simulink model "TestRtrIkslx"  (R2020a)
settings: Solver=VariableStepAuto  StartTime=0.0  StopTime=10.0  RelTol=1e-3
values from neighbouring files (symbols this model uses):
  l2 = 0.3    [TestingIkRTR.m]    (also in TestingScriptRTR.m)
  l3 = 0.2    [TestingIkRTR.m]    (also in TestingScriptRTR.m)
settings Model: Creator=ja  LastModifiedBy=ja

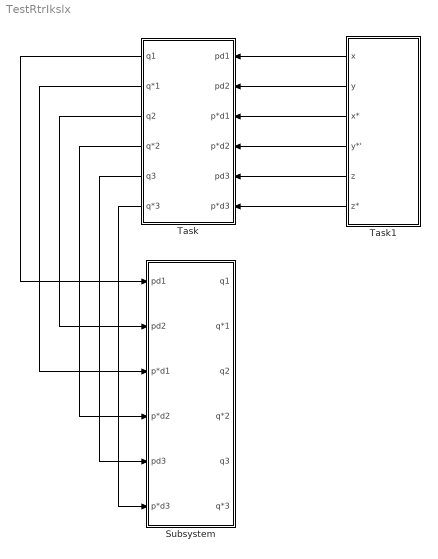
== system TestRtrIkslx ==
  Subsystem : Subsystem
  Task : Subsystem
  Task1 : Subsystem
  wires:
  Task1/5(z) -> Task/5(pd3)
  Task1/6(z*) -> Task/6(p*d3)
  Task1/1(x) -> Task/1(pd1)
  Task1/2(y) -> Task/2(pd2)
  Task1/3(x*) -> Task/3(p*d1)
  Task1/4(y*') -> Task/4(p*d2)
  Task/1(q1) -> Subsystem/1(pd1)
  Task/3(q2) -> Subsystem/2(pd2)
  Task/2(q*1) -> Subsystem/3(p*d1)
  Task/4(q*2) -> Subsystem/4(p*d2)
  Task/5(q3) -> Subsystem/5(pd3)
  Task/6(q*3) -> Subsystem/6(p*d3)

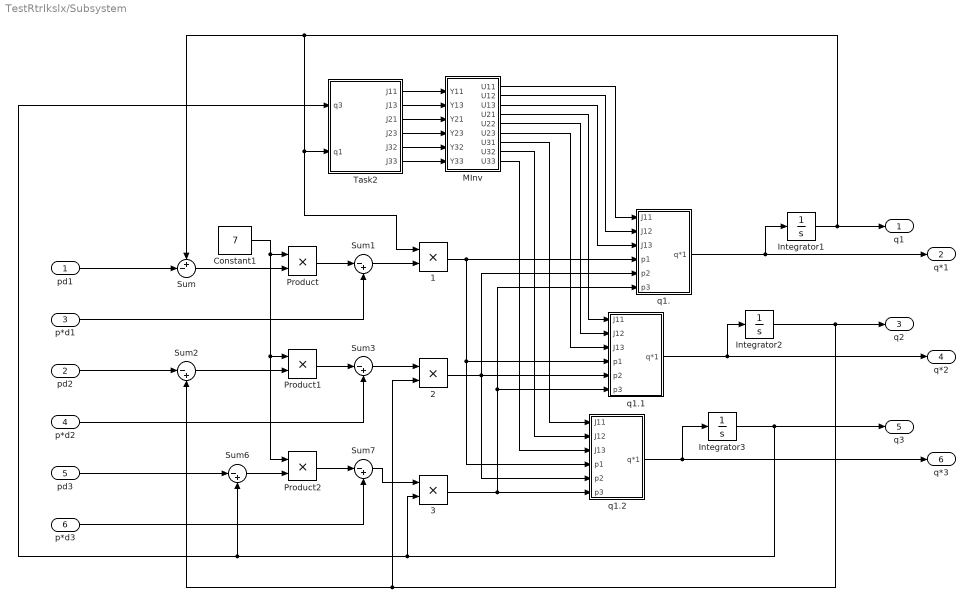
== system TestRtrIkslx/Subsystem ==
  pd1 : Inport
  pd2 : Inport  Port=2
  p*d1 : Inport  Port=3
  p*d2 : Inport  Port=4
  pd3 : Inport  Port=5
  p*d3 : Inport  Port=6
  1 : Product
  2 : Product
  3 : Product
  Constant1 : Constant  Value=7
  Integrator1 : Integrator
  Integrator2 : Integrator
  Integrator3 : Integrator  InitialCondition=0.1
  MInv : MATLAB Function  TreatAsAtomicUnit=on
  Product : Product
  Product1 : Product
  Product2 : Product
  Sum : Sum  Inputs=+-|
  Sum{1..3,6..7} (5 alike) : Sum  Inputs=|-+
  Task2 : Subsystem
  q1. : Subsystem
  q1.1 : Subsystem
  q1.2 : Subsystem
  q1 : Outport
  q*1 : Outport  Port=2
  q2 : Outport  Port=3
  q*2 : Outport  Port=4
  q3 : Outport  Port=5
  q*3 : Outport  Port=6
  wires:
  Task2/1(J11) -> MInv/1(Y11)
  Sum/1 -> Product/2
  q1.1/1(q*1) -> q*2/1, Integrator2/1
  Integrator1/1 -> q1/1, Sum/1, 1/1, Task2/2(q1)
  pd3/1 -> Sum6/1
  MInv/7(U31) -> q1.2/1(J11)
  p*d3/1 -> Sum7/2
  MInv/3(U13) -> q1./3(J13)
  MInv/4(U21) -> q1.1/1(J11)
  Product/1 -> Sum1/1
  2/1 -> q1.2/5(p2), q1.1/5(p2), q1./5(p2)
  q1./1(q*1) -> q*1/1, Integrator1/1
  MInv/5(U22) -> q1.1/2(J12)
  p*d2/1 -> Sum3/2
  Integrator3/1 -> q3/1, 3/2, Task2/1(q3), Sum6/2
  Task2/3(J21) -> MInv/3(Y21)
  Constant1/1 -> Product2/1, Product1/1, Product/1
  MInv/8(U32) -> q1.2/2(J12)
  q1.2/1(q*1) -> q*3/1, Integrator3/1
  MInv/9(U33) -> q1.2/3(J13)
  MInv/2(U12) -> q1./2(J12)
  Sum7/1 -> 3/1
  Task2/6(J33) -> MInv/6(Y33)
  Task2/4(J23) -> MInv/4(Y23)
  1/1 -> q1./4(p1), q1.2/4(p1), q1.1/4(p1)
  MInv/6(U23) -> q1.1/3(J13)
  Task2/5(J32) -> MInv/5(Y32)
  p*d1/1 -> Sum1/2
  Product2/1 -> Sum7/1
  pd2/1 -> Sum2/1
  MInv/1(U11) -> q1./1(J11)
  pd1/1 -> Sum/2
  Sum2/1 -> Product1/2
  Sum6/1 -> Product2/2
  Integrator2/1 -> q2/1, Sum2/2, 2/2
  Sum1/1 -> 1/2
  3/1 -> q1./6(p3), q1.1/6(p3), q1.2/6(p3)
  Sum3/1 -> 2/1
  Task2/2(J13) -> MInv/2(Y13)
  Product1/1 -> Sum3/1

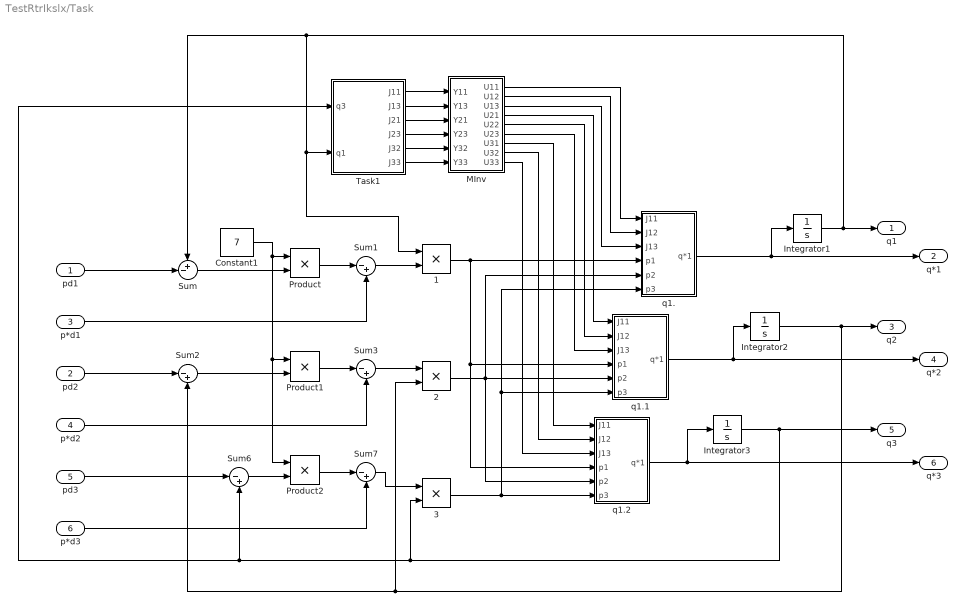
== system TestRtrIkslx/Task ==
  pd1 : Inport
  pd2 : Inport  Port=2
  p*d1 : Inport  Port=3
  p*d2 : Inport  Port=4
  pd3 : Inport  Port=5
  p*d3 : Inport  Port=6
  1 : Product
  2 : Product
  3 : Product
  Constant1 : Constant  Value=7
  Integrator1 : Integrator
  Integrator2 : Integrator
  Integrator3 : Integrator  InitialCondition=0.1
  MInv : MATLAB Function  TreatAsAtomicUnit=on
  Product : Product
  Product1 : Product
  Product2 : Product
  Sum : Sum  Inputs=+-|
  Sum{1..3,6..7} (5 alike) : Sum  Inputs=|-+
  Task1 : Subsystem
  q1. : Subsystem
  q1.1 : Subsystem
  q1.2 : Subsystem
  q1 : Outport
  q*1 : Outport  Port=2
  q2 : Outport  Port=3
  q*2 : Outport  Port=4
  q3 : Outport  Port=5
  q*3 : Outport  Port=6
  wires:
  pd1/1 -> Sum/2
  Sum1/1 -> 1/2
  Product/1 -> Sum1/1
  Product1/1 -> Sum3/1
  Sum/1 -> Product/2
  Integrator1/1 -> q1/1, Sum/1, 1/1, Task1/2(q1)
  p*d2/1 -> Sum3/2
  Sum2/1 -> Product1/2
  Integrator2/1 -> q2/1, Sum2/2, 2/2
  pd2/1 -> Sum2/1
  p*d1/1 -> Sum1/2
  Sum3/1 -> 2/1
  Sum6/1 -> Product2/2
  pd3/1 -> Sum6/1
  Constant1/1 -> Product2/1, Product1/1, Product/1
  p*d3/1 -> Sum7/2
  Product2/1 -> Sum7/1
  Sum7/1 -> 3/1
  Task1/1(J11) -> MInv/1(Y11)
  Task1/2(J13) -> MInv/2(Y13)
  Task1/3(J21) -> MInv/3(Y21)
  Task1/4(J23) -> MInv/4(Y23)
  Task1/5(J32) -> MInv/5(Y32)
  Task1/6(J33) -> MInv/6(Y33)
  1/1 -> q1./4(p1), q1.2/4(p1), q1.1/4(p1)
  2/1 -> q1.2/5(p2), q1.1/5(p2), q1./5(p2)
  3/1 -> q1./6(p3), q1.1/6(p3), q1.2/6(p3)
  MInv/1(U11) -> q1./1(J11)
  MInv/2(U12) -> q1./2(J12)
  MInv/3(U13) -> q1./3(J13)
  MInv/4(U21) -> q1.1/1(J11)
  MInv/5(U22) -> q1.1/2(J12)
  MInv/6(U23) -> q1.1/3(J13)
  MInv/7(U31) -> q1.2/1(J11)
  MInv/8(U32) -> q1.2/2(J12)
  MInv/9(U33) -> q1.2/3(J13)
  Integrator3/1 -> q3/1, 3/2, Task1/1(q3), Sum6/2
  q1./1(q*1) -> Integrator1/1, q*1/1
  q1.1/1(q*1) -> Integrator2/1, q*2/1
  q1.2/1(q*1) -> Integrator3/1, q*3/1

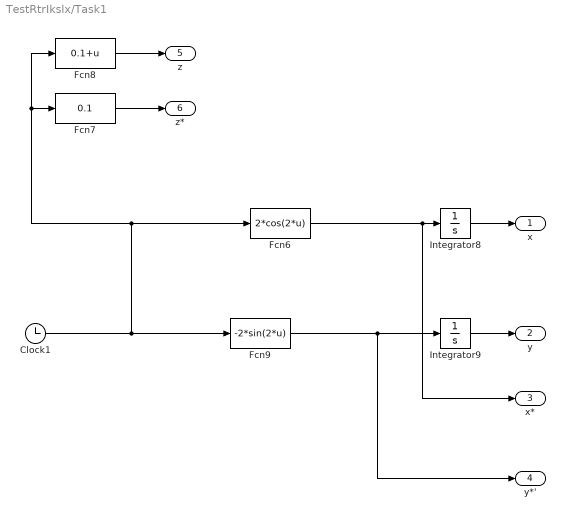
== system TestRtrIkslx/Task1 ==
  Clock1 : Clock
  Fcn6 : Fcn  Expr=2*cos(2*u)
  Fcn7 : Fcn  Expr=0.1
  Fcn8 : Fcn  Expr=0.1+u
  Fcn9 : Fcn  Expr=-2*sin(2*u)
  Integrator8 : Integrator
  Integrator9 : Integrator  InitialCondition=1
  x : Outport
  y : Outport  Port=2
  x* : Outport  Port=3
  y*' : Outport  Port=4
  z : Outport  Port=5
  z* : Outport  Port=6
  wires:
  Fcn8/1 -> z/1
  Fcn7/1 -> z*/1
  Integrator8/1 -> x/1
  Fcn6/1 -> x*/1, Integrator8/1
  Clock1/1 -> Fcn8/1, Fcn7/1, Fcn6/1, Fcn9/1
  Integrator9/1 -> y/1
  Fcn9/1 -> y*'/1, Integrator9/1

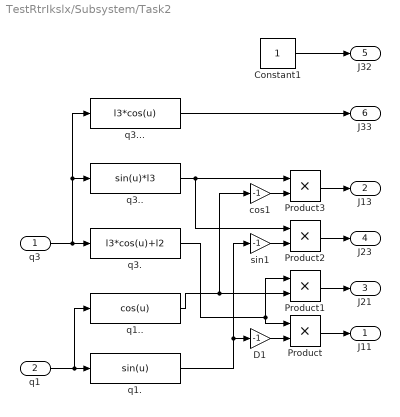
== system TestRtrIkslx/Subsystem/Task2 ==
  q3 : Inport
  q1 : Inport  Port=2
  Constant1 : Constant
  D1 : Gain  Gain=-1
  Product{,1..3} (4 alike) : Product
  cos1 : Gain  Gain=-1
  q1. : Fcn  Expr=sin(u)
  q1.. : Fcn  Expr=cos(u)
  q3. : Fcn  Expr=l3*cos(u)+l2
  q3.. : Fcn  Expr=sin(u)*l3
  q3... : Fcn  Expr=l3*cos(u)
  sin1 : Gain  Gain=-1
  J11 : Outport
  J13 : Outport  Port=2
  J21 : Outport  Port=3
  J23 : Outport  Port=4
  J32 : Outport  Port=5
  J33 : Outport  Port=6
  wires:
  q3/1 -> q3.../1, q3../1, q3./1
  q1/1 -> q1../1, q1./1
  q3./1 -> Product/1, Product1/1
  Product/1 -> J11/1
  D1/1 -> Product/2
  q1./1 -> sin1/1, D1/1
  q1../1 -> cos1/1, Product1/2
  q3../1 -> Product2/1, Product3/1
  sin1/1 -> Product2/2
  cos1/1 -> Product3/2
  Product3/1 -> J13/1
  Product1/1 -> J21/1
  Product2/1 -> J23/1
  q3.../1 -> J33/1
  Constant1/1 -> J32/1

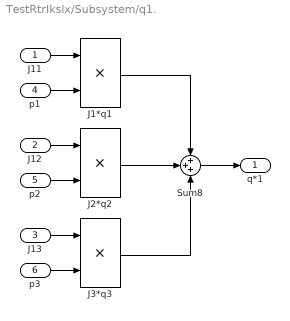
== system TestRtrIkslx/Subsystem/q1. ==
  J11 : Inport
  J12 : Inport  Port=2
  J13 : Inport  Port=3
  p1 : Inport  Port=4
  p2 : Inport  Port=5
  p3 : Inport  Port=6
  J1*q1 : Product
  J2*q2 : Product
  J3*q3 : Product
  Sum8 : Sum  Inputs=+++
  q*1 : Outport
  wires:
  J11/1 -> J1*q1/1
  p1/1 -> J1*q1/2
  J12/1 -> J2*q2/1
  J13/1 -> J3*q3/1
  p2/1 -> J2*q2/2
  p3/1 -> J3*q3/2
  J2*q2/1 -> Sum8/2
  J1*q1/1 -> Sum8/1
  J3*q3/1 -> Sum8/3
  Sum8/1 -> q*1/1

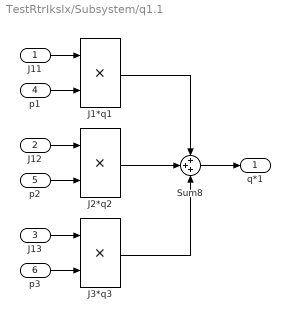
== system TestRtrIkslx/Subsystem/q1.1 ==
  J11 : Inport
  J12 : Inport  Port=2
  J13 : Inport  Port=3
  p1 : Inport  Port=4
  p2 : Inport  Port=5
  p3 : Inport  Port=6
  J1*q1 : Product
  J2*q2 : Product
  J3*q3 : Product
  Sum8 : Sum  Inputs=+++
  q*1 : Outport
  wires:
  J11/1 -> J1*q1/1
  p1/1 -> J1*q1/2
  J12/1 -> J2*q2/1
  J13/1 -> J3*q3/1
  p2/1 -> J2*q2/2
  p3/1 -> J3*q3/2
  J2*q2/1 -> Sum8/2
  J1*q1/1 -> Sum8/1
  J3*q3/1 -> Sum8/3
  Sum8/1 -> q*1/1

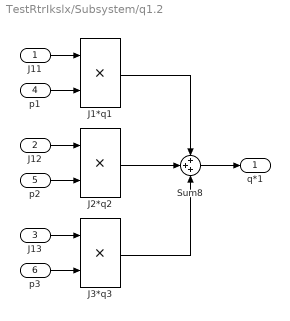
== system TestRtrIkslx/Subsystem/q1.2 ==
  J11 : Inport
  J12 : Inport  Port=2
  J13 : Inport  Port=3
  p1 : Inport  Port=4
  p2 : Inport  Port=5
  p3 : Inport  Port=6
  J1*q1 : Product
  J2*q2 : Product
  J3*q3 : Product
  Sum8 : Sum  Inputs=+++
  q*1 : Outport
  wires:
  J11/1 -> J1*q1/1
  p1/1 -> J1*q1/2
  J12/1 -> J2*q2/1
  J13/1 -> J3*q3/1
  p2/1 -> J2*q2/2
  p3/1 -> J3*q3/2
  J2*q2/1 -> Sum8/2
  J1*q1/1 -> Sum8/1
  J3*q3/1 -> Sum8/3
  Sum8/1 -> q*1/1

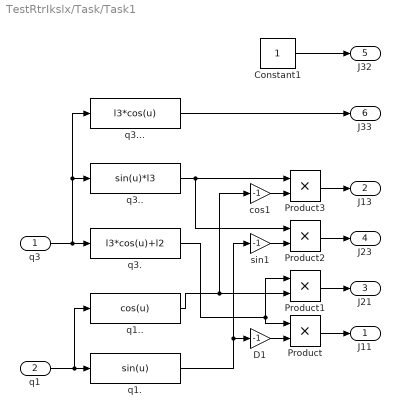
== system TestRtrIkslx/Task/Task1 ==
  q3 : Inport
  q1 : Inport  Port=2
  Constant1 : Constant
  D1 : Gain  Gain=-1
  Product{,1..3} (4 alike) : Product
  cos1 : Gain  Gain=-1
  q1. : Fcn  Expr=sin(u)
  q1.. : Fcn  Expr=cos(u)
  q3. : Fcn  Expr=l3*cos(u)+l2
  q3.. : Fcn  Expr=sin(u)*l3
  q3... : Fcn  Expr=l3*cos(u)
  sin1 : Gain  Gain=-1
  J11 : Outport
  J13 : Outport  Port=2
  J21 : Outport  Port=3
  J23 : Outport  Port=4
  J32 : Outport  Port=5
  J33 : Outport  Port=6
  wires:
  q3/1 -> q3.../1, q3../1, q3./1
  q1/1 -> q1../1, q1./1
  q3./1 -> Product/1, Product1/1
  Product/1 -> J11/1
  D1/1 -> Product/2
  q1./1 -> sin1/1, D1/1
  q1../1 -> cos1/1, Product1/2
  q3../1 -> Product2/1, Product3/1
  sin1/1 -> Product2/2
  cos1/1 -> Product3/2
  Product3/1 -> J13/1
  Product1/1 -> J21/1
  Product2/1 -> J23/1
  q3.../1 -> J33/1
  Constant1/1 -> J32/1

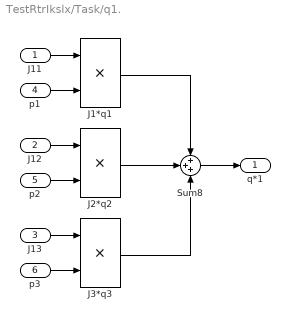
== system TestRtrIkslx/Task/q1. ==
  J11 : Inport
  J12 : Inport  Port=2
  J13 : Inport  Port=3
  p1 : Inport  Port=4
  p2 : Inport  Port=5
  p3 : Inport  Port=6
  J1*q1 : Product
  J2*q2 : Product
  J3*q3 : Product
  Sum8 : Sum  Inputs=+++
  q*1 : Outport
  wires:
  J11/1 -> J1*q1/1
  p1/1 -> J1*q1/2
  J12/1 -> J2*q2/1
  J13/1 -> J3*q3/1
  p2/1 -> J2*q2/2
  p3/1 -> J3*q3/2
  J2*q2/1 -> Sum8/2
  J1*q1/1 -> Sum8/1
  J3*q3/1 -> Sum8/3
  Sum8/1 -> q*1/1

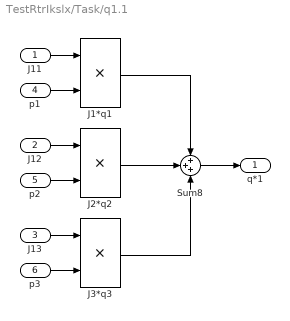
== system TestRtrIkslx/Task/q1.1 ==
  J11 : Inport
  J12 : Inport  Port=2
  J13 : Inport  Port=3
  p1 : Inport  Port=4
  p2 : Inport  Port=5
  p3 : Inport  Port=6
  J1*q1 : Product
  J2*q2 : Product
  J3*q3 : Product
  Sum8 : Sum  Inputs=+++
  q*1 : Outport
  wires:
  J11/1 -> J1*q1/1
  p1/1 -> J1*q1/2
  J12/1 -> J2*q2/1
  J13/1 -> J3*q3/1
  p2/1 -> J2*q2/2
  p3/1 -> J3*q3/2
  J2*q2/1 -> Sum8/2
  J1*q1/1 -> Sum8/1
  J3*q3/1 -> Sum8/3
  Sum8/1 -> q*1/1

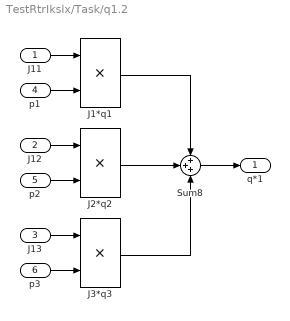
== system TestRtrIkslx/Task/q1.2 ==
  J11 : Inport
  J12 : Inport  Port=2
  J13 : Inport  Port=3
  p1 : Inport  Port=4
  p2 : Inport  Port=5
  p3 : Inport  Port=6
  J1*q1 : Product
  J2*q2 : Product
  J3*q3 : Product
  Sum8 : Sum  Inputs=+++
  q*1 : Outport
  wires:
  J11/1 -> J1*q1/1
  p1/1 -> J1*q1/2
  J12/1 -> J2*q2/1
  J13/1 -> J3*q3/1
  p2/1 -> J2*q2/2
  p3/1 -> J3*q3/2
  J2*q2/1 -> Sum8/2
  J1*q1/1 -> Sum8/1
  J3*q3/1 -> Sum8/3
  Sum8/1 -> q*1/1

== matlab function TestRtrIkslx/Subsystem/MInv ==
  data: Y11 input; Y13 input; Y21 input; Y23 input; Y32 input; U11 output; U12 output; U13 output; Y33 input; U21 output; U22 output; U23 output; U31 output; U32 output; U33 output
function [U11, U12, U13, U21, U22, U23, U31, U32, U33] = c(Y11, Y13, Y21, Y23, Y32, Y33)

M = [Y11 0 Y13; Y21 0 Y23; 0 Y32 Y33];
F = inv(M);

U11 = F(1);
U12 = F(2);
U13 = F(3);
U21 = F(4);
U22 = F(5);
U23 = F(6);
U31 = F(7);
U32 = F(9);
U33 = F(9);

== matlab function TestRtrIkslx/Task/MInv ==
  data: Y11 input; Y13 input; Y21 input; Y23 input; Y32 input; U11 output; U12 output; U13 output; Y33 input; U21 output; U22 output; U23 output; U31 output; U32 output; U33 output
function [U11, U12, U13, U21, U22, U23, U31, U32, U33] = c(Y11, Y13, Y21, Y23, Y32, Y33)

M = [Y11 0 Y13; Y21 0 Y23; 0 Y32 Y33];
F = inv(M);

U11 = F(1);
U12 = F(2);
U13 = F(3);
U21 = F(4);
U22 = F(5);
U23 = F(6);
U31 = F(7);
U32 = F(9);
U33 = F(9);
